simulink model "task9b_v24"  (R2024a)
settings: Solver=VariableStepAuto  StartTime=0.0  StopTime=3  RelTol=1e-3
values from neighbouring files (symbols this model uses):
  tInterval = [0 5]    [task7b.m]    (also in task7b2.m; task8b_setup.m = [0 10]; task9_visu.m = [0 10]; task9b_setup.m = [0 10])
undefined symbols (not defined in the file or in its folder): eul2tform, trvec2tform
libraries: robotcorelib x5, robotmaniplib x2
settings Model: Creator=laith  LastModifiedBy=laith

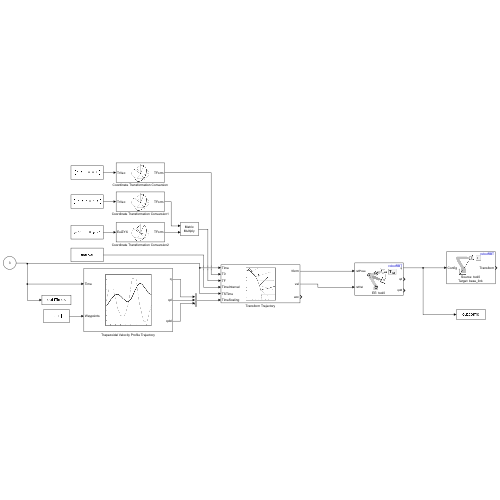
[thumbnail: Simulink's stored preview of the top-level diagram]
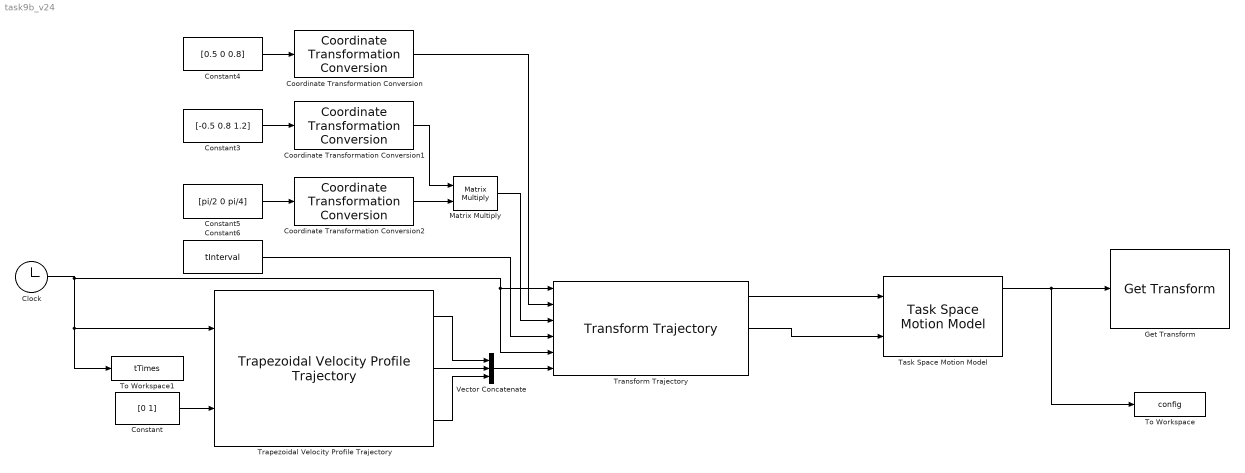
== system task9b_v24 ==
  Clock : Clock
      settings: Decimation=100
  Constant : Constant  Value=[0 1]  VectorParams1D=off
  Constant3 : Constant  Value=[-0.5 0.8 1.2]
  Constant4 : Constant  Value=[0.5 0 0.8]
  Constant5 : Constant  Value=[pi/2 0 pi/4]
  Constant6 : Constant  Value=tInterval
  Coordinate Transformation Conversion : robotcorelib/Coordinate Transformation Conversion  InputRepresentation=Translation Vector  InputEulerSequence=ZYX  ShowTrVecInputPort=on  OutputRepresentation=Homogeneous Transformation  OutputEulerSequence=ZYX  ShowTrVecOutputPort=on  SimulateUsing=Interpreted execution
  Coordinate Transformation Conversion1 : robotcorelib/Coordinate Transformation Conversion  InputRepresentation=Translation Vector  InputEulerSequence=ZYX  ShowTrVecInputPort=on  OutputRepresentation=Homogeneous Transformation  OutputEulerSequence=ZYX  ShowTrVecOutputPort=off  SimulateUsing=Interpreted execution
  Coordinate Transformation Conversion2 : robotcorelib/Coordinate Transformation Conversion  InputRepresentation=Euler Angles  InputEulerSequence=ZYX  ShowTrVecInputPort=off  OutputRepresentation=Homogeneous Transformation  OutputEulerSequence=ZYX  ShowTrVecOutputPort=on  SimulateUsing=Interpreted execution
  Get Transform : robotmaniplib/Get Transform  RigidBodyTree=robotRBT  SourceBody=tool0  TargetBody=base_link  SimulateUsing=Interpreted execution
  Matrix Multiply : Product  Multiplication=Matrix(*)
  Task Space Motion Model : robotmaniplib/Task Space Motion Model  RigidBodyTree=robotRBT  EndEffector=tool0  ProportionalGain=500*eye(6)  DerivativeGain=100*eye(6)  JointDamping=1  ShowExternalForcePort=off  InitConfig=homeConfig.JointPosition  InitJointVel=0  SimulateUsing=Interpreted execution
  To Workspace : ToWorkspace  VariableName=config  SampleTime=-1
  To Workspace1 : ToWorkspace  VariableName=tTimes  SampleTime=-1
  Transform Trajectory : robotcorelib/Transform Trajectory  WaypointSource=External  T0=trvec2tform( [ 1, 10, -1 ] )  TF=eul2tform( [ 0, pi, pi / 2 ] )  TimeInterval=[ 2, 3 ]  CustomTimeScaling=on  ParameterSource=External  TSTime=2:0.1:3  TimeScaling=[ 0:0.1:1; ones( 1, 11 ); zeros( 1, 11 ) ]  SimulateUsing=Interpreted execution
      settings: LibrarySourceBlock=robotutilslib/Transform Trajectory
  Trapezoidal Velocity Profile Trajectory : robotcorelib/Trapezoidal Velocity Profile Trajectory  WaypointSource=External  Waypoints=[ 0, -0.5, -1; 0, 0.5, 1 ]  NumParams=0  Parameter1=End Time  Parameter2=End Time  ParameterSource=External  PeakVelocity=[ 2; 2 ]  Acceleration=[ 1; 2 ]  EndTime=[ 1; 1 ]  AccelTime=[ 1; 2 ]  SimulateUsing=Code generation
  Vector Concatenate : Concatenate  NumInputs=3  Mode=Multidimensional array
  wires:
  Matrix Multiply/1 -> Transform Trajectory/3
  Trapezoidal Velocity Profile Trajectory/3 -> Vector Concatenate/3
  Constant6/1 -> Transform Trajectory/4
  Constant/1 -> Trapezoidal Velocity Profile Trajectory/2
  Coordinate Transformation Conversion2/1 -> Matrix Multiply/2
  Coordinate Transformation Conversion1/1 -> Matrix Multiply/1
  Vector Concatenate/1 -> Transform Trajectory/6
  Trapezoidal Velocity Profile Trajectory/2 -> Vector Concatenate/2
  Trapezoidal Velocity Profile Trajectory/1 -> Vector Concatenate/1
  Coordinate Transformation Conversion/1 -> Transform Trajectory/2
  Constant4/1 -> Coordinate Transformation Conversion/1
  Constant5/1 -> Coordinate Transformation Conversion2/1
  Clock/1 -> To Workspace1/1, Trapezoidal Velocity Profile Trajectory/1, Transform Trajectory/1, Transform Trajectory/5
  Constant3/1 -> Coordinate Transformation Conversion1/1
  Task Space Motion Model/1 -> To Workspace/1, Get Transform/1
  Transform Trajectory/1 -> Task Space Motion Model/1
  Transform Trajectory/2 -> Task Space Motion Model/2
